simulink model "DC_DC_converters"  (Simulink 10.3)
settings: Solver=ode4  StartTime=0.0  StopTime=.15  FixedStep=Ts  MaxStep=1e-4  RelTol=1e-3
undefined symbols (not defined in the file): Ts
libraries: spsSeriesRLCBranchLib x3, spsVoltageMeasurementLib x3, spsCurrentMeasurementLib x2, spsDCVoltageSourceLib x2, spsDiodeLib x1, spsGroundLib x1, spsMeanLib x1, spsMosfetLib x1, spsPWMGeneratorDCDCLib x1, spsRMSLib x1
settings Model: Creator=D  LastModifiedBy=Ayush Jindal  MultithreadedSim=on
settings DataIOCC: LimitDataPoints=on  SaveFormat=StructureWithTime  SignalLoggingSaveFormat=Dataset
settings OptimizationCC: ExpressionDepthLimit=128
settings DebuggingCC: UnderspecifiedInitializationDetection=Simplified  MergeDetectMultiDrivingBlocksExec=error  FcnCallInpInsideContextMsg=error  StateNameClashWarn=none
settings HardwareCC: ProdBitPerPointer=64  ProdLargestAtomicFloat=Float  ProdIntDivRoundTo=Zero  ProdEndianess=LittleEndian  ProdHWDeviceType=Specified
settings GRTTargetCC: CombineOutputUpdateFcns=on  GRTInterface=off
settings ConfigComp: CovSFcnEnable=off
settings SimscapeCC: SimscapeNormalizeSystem=off

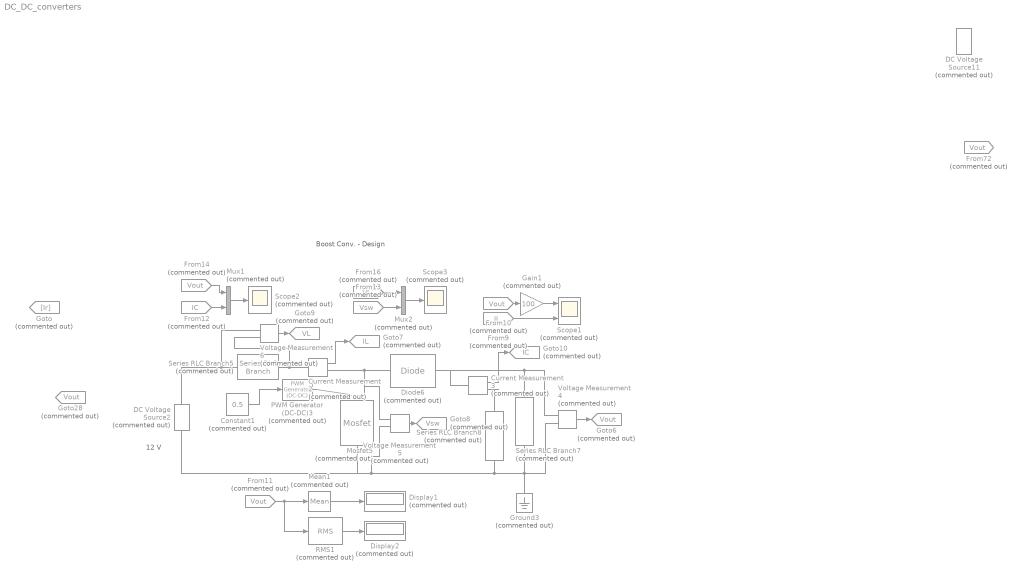
== system DC_DC_converters ==
  note: 12 V
  note: Boost Conv. - Design
  Constant1 : Constant  Commented=on  Value=0.5
  Current Measurement2 : spsCurrentMeasurementLib/Current Measurement  Commented=on  PhasorSimulation=off  OutputType=Complex  PSBequivalent=0
  Current Measurement3 : spsCurrentMeasurementLib/Current Measurement  Commented=on  PhasorSimulation=off  OutputType=Complex  PSBequivalent=0
  DC Voltage Source11 : spsDCVoltageSourceLib/DC Voltage Source  Commented=on  Amplitude=24  Measurements=None
  DC Voltage Source2 : spsDCVoltageSourceLib/DC Voltage Source  Commented=on  Amplitude=12  Measurements=None
  Diode6 : spsDiodeLib/Diode  Commented=on  Ron=1e-7  Lon=0  Vf=0  IC=0  UseSnubber=0  Rs=1e6  Cs=1e6  Measurements=off
  Display1 : Display  Commented=on
  Display2 : Display  Commented=on
  From{10..11,14,72} (4 alike) : From  Commented=on  GotoTag=Vout  TagVisibility=global
  From12 : From  Commented=on  GotoTag=IC  TagVisibility=global
  From13 : From  Commented=on  GotoTag=Vsw  TagVisibility=global
  From16 : From  Commented=on  GotoTag=VL  TagVisibility=global
  From9 : From  Commented=on  GotoTag=IL  TagVisibility=global
  Gain1 : Gain  Commented=on  Gain=100
  Goto : Goto  Commented=on  GotoTag=Ir
  Goto10 : Goto  Commented=on  GotoTag=IC  TagVisibility=global
  Goto28 : Goto  Commented=on  GotoTag=Vout  TagVisibility=global
  Goto6 : Goto  Commented=on  GotoTag=Vout  TagVisibility=global
  Goto7 : Goto  Commented=on  GotoTag=IL  TagVisibility=global
  Goto8 : Goto  Commented=on  GotoTag=Vsw  TagVisibility=global
  Goto9 : Goto  Commented=on  GotoTag=VL  TagVisibility=global
  Ground3 : spsGroundLib/Ground  Commented=on  LConnTagsString=a
  Mean1 : spsMeanLib/Mean  Commented=on  Freq=5000  Vinit=0  Ts=0
  Mosfet5 : spsMosfetLib/Mosfet  Commented=on  Ron=1e-7  Lon=0  Rd=1e-10  Vfd=0  IC=0  Rs=inf  Cs=0  Measurements=off
  Mux1 : Mux  Commented=on  Inputs=2
  Mux2 : Mux  Commented=on  Inputs=2
  PWM Generator (DC-DC)3 : spsPWMGeneratorDCDCLib/PWM Generator (DC-DC)  Commented=on  Fsw=10000  Ts=Ts
  RMS1 : spsRMSLib/RMS  Commented=on  TrueRMS=on  Freq=10000  RMSInit=0  Ts=0
  Scope1 : Scope  Commented=on  NumInputPorts=2
  Scope2 : Scope  Commented=on
  Scope3 : Scope  Commented=on
  Series RLC Branch5 : spsSeriesRLCBranchLib/Series RLC Branch  Commented=on  LConnTagsString=__new0  RConnTagsString=__new0  BranchType=L  Resistance=0.000001  Inductance=0.0015  SetiL0=off  InitialCurrent=0  Capacitance=1e-6  Setx0=off  InitialVoltage=0  Measurements=None
  Series RLC Branch7 : spsSeriesRLCBranchLib/Series RLC Branch  Commented=on  LConnTagsString=__new0  RConnTagsString=__new0  BranchType=R  Resistance=12  Inductance=1e-3  SetiL0=off  InitialCurrent=0  Capacitance=1000e-6  Setx0=on  InitialVoltage=800  Measurements=None
  Series RLC Branch8 : spsSeriesRLCBranchLib/Series RLC Branch  Commented=on  LConnTagsString=__new0  RConnTagsString=__new0  BranchType=C  Resistance=6  Inductance=1e-3  SetiL0=off  InitialCurrent=0  Capacitance=416.67e-6  Setx0=off  InitialVoltage=800  Measurements=None
  Voltage Measurement4 : spsVoltageMeasurementLib/Voltage Measurement  Commented=on  PhasorSimulation=off  OutputType=Complex  PSBequivalent=0
  Voltage Measurement5 : spsVoltageMeasurementLib/Voltage Measurement  Commented=on  PhasorSimulation=off  OutputType=Complex  PSBequivalent=0
  Voltage Measurement6 : spsVoltageMeasurementLib/Voltage Measurement  Commented=on  PhasorSimulation=off  OutputType=Complex  PSBequivalent=0
  wires:
  Mux1/1 -> Scope2/1
  From12/1 -> Mux1/2
  Current Measurement2/1 -> Goto7/1
  RMS1/1 -> Display2/1
  Constant1/1 -> PWM Generator (DC-DC)3/1
  From14/1 -> Mux1/1
  Mean1/1 -> Display1/1
  From9/1 -> Scope1/2
  Voltage Measurement4/1 -> Goto6/1
  Voltage Measurement5/1 -> Goto8/1
  Gain1/1 -> Scope1/1
  From11/1 -> RMS1/1, Mean1/1
  PWM Generator (DC-DC)3/1 -> Mosfet5/1
  From10/1 -> Gain1/1
  From13/1 -> Mux2/2
  From16/1 -> Mux2/1
  Mux2/1 -> Scope3/1
  Voltage Measurement6/1 -> Goto9/1
  Current Measurement3/1 -> Goto10/1
  ? -> Goto28/1
  connections:
  Series RLC Branch7/LConn1 -- Current Measurement3/LConn1 -- Diode6/RConn1 -- Voltage Measurement4/LConn1
  Voltage Measurement4/LConn2 -- Ground3/LConn1 -- Series RLC Branch7/RConn1 -- DC Voltage Source2/LConn1 -- Mosfet5/RConn1 -- Voltage Measurement5/LConn2 -- Series RLC Branch8/RConn1
  DC Voltage Source2/RConn1 -- Voltage Measurement6/LConn1 -- Series RLC Branch5/LConn1
  Current Measurement2/LConn1 -- Voltage Measurement6/LConn2 -- Series RLC Branch5/RConn1
  Current Measurement2/RConn1 -- Diode6/LConn1 -- Mosfet5/LConn1 -- Voltage Measurement5/LConn1
  Current Measurement3/RConn1 -- Series RLC Branch8/LConn1
